simulink subsystem "SignalSelector"  (R2024a)
settings: Solver=VariableStepAuto  StartTime=0.0  StopTime=10.0  RelTol=1e-3
model mask{st=Step, Amp=0, dt=0, RiseT=0}
  mask prompts: st "Signal Type"; Amp "Amplitute"; dt "Delay Time"; RiseT "Rise Time"
settings Model: Creator=leofong  LastModifiedBy=leofong

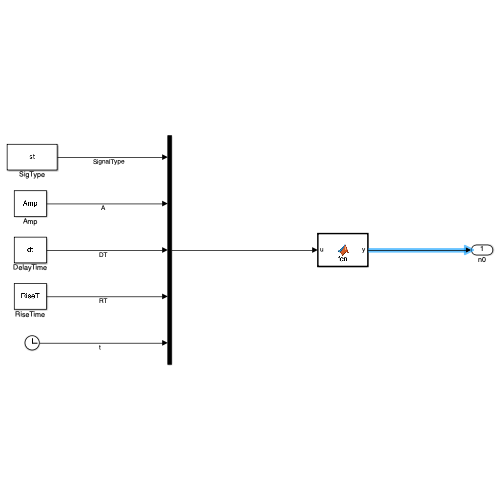
[thumbnail: Simulink's stored preview of the top-level diagram]
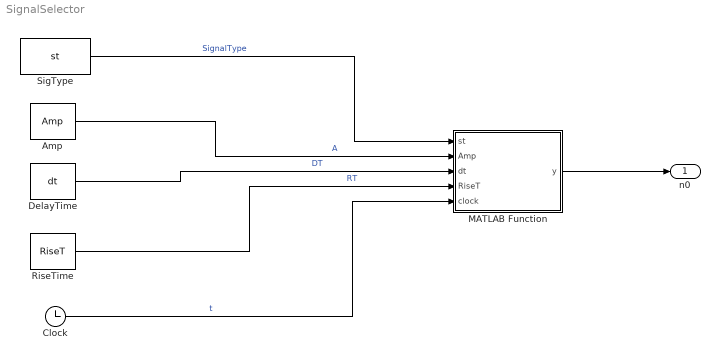
== system SignalSelector ==
  Amp : Constant  Value=Amp
  Clock : Clock
  DelayTime : Constant  Value=dt
  MATLAB Function : MATLAB Function  TreatAsAtomicUnit=on
  RiseTime : Constant  Value=RiseT
  SigType : Constant  Value=st
  n0 : Outport
  wires:
  MATLAB Function/1(y) -> n0/1
  Clock/1 -> MATLAB Function/5(clock)  "t"
  SigType/1 -> MATLAB Function/1(st)  "SignalType"
  Amp/1 -> MATLAB Function/2(Amp)  "A"
  DelayTime/1 -> MATLAB Function/3(dt)  "DT"
  RiseTime/1 -> MATLAB Function/4(RiseT)  "RT"

== matlab function SignalSelector/MATLAB Function ==
  data: st input; y output; Amp input; dt input; RiseT input; clock input
function y = fcn(st,Amp,dt,RiseT,clock)
    switch st
        case 1
            if clock > dt
                y = Amp;
            else
                y = 0;
            end
        case 2
            y = min(Amp,clock/RiseT);
        case 3
            y = Amp/(1+exp(-clock + RiseT/2));
        otherwise
            y = 0;
    end
end


% y = self;
